simulink model "Simulink1potradi2"  (R2017b)
settings: Solver=VariableStepAuto  StartTime=0  StopTime=200  MinStep=0.1  RelTol=1e-3
values from neighbouring files (symbols this model uses):
  A = [0 1 1 1 ... (first row only)    [Initial.m]    (also in matlab_promjena_form.mat = [0 1 1 1 1 1 0 1 1 1 1 1 ... (25 elements, 5x5)])
  c_d = 2.5    [ardrone_params.m]    (also in matlab_promjena_form.mat)
  g = 9.81    [ardrone_params.m]    (also in matlab_promjena_form.mat)
  m = 1.65    [ardrone_params.m]    (also in matlab_promjena_form.mat)
  pitch_max = 0.4    [ardrone_params.m]    (also in matlab_promjena_form.mat)
  R1 = [0  -1  -1  -2  -2; 0  1  -1  2  -2]    [matlab_promjena_form.mat]
  R2 = [0,0,0,0; -1, 1, -3, 3]    [Initial.m]    (also in matlab_promjena_form.mat = [9  7  5  3  1; 0  0  0  0  0])
  roll_max = 0.4    [ardrone_params.m]    (also in matlab_promjena_form.mat)
  T_pitch = 0.4    [ardrone_params.m]    (also in matlab_promjena_form.mat)
  T_roll = 0.4    [ardrone_params.m]    (also in matlab_promjena_form.mat)
  T_yaw = 0.8    [ardrone_params.m]    (also in matlab_promjena_form.mat)
  T_z = 0.6    [ardrone_params.m]    (also in matlab_promjena_form.mat)
  x0 = [20, 60, 30, 50]    [Initial.m]    (also in matlab_promjena_form.mat = [0 -1 -1 -2 -2])
  y0 = [60, 20, 50, 30]    [Initial.m]    (also in matlab_promjena_form.mat = [0 1 -1 2 -2])
  yaw_rate_max = 0.7864    [ardrone_params.m]    (also in matlab_promjena_form.mat)
  z_rate_max = 0.7    [ardrone_params.m]    (also in matlab_promjena_form.mat)
settings Model: Creator=Mare  LastModifiedBy=Mare
settings SolverCC: ZeroCrossAlgorithm=Adaptive

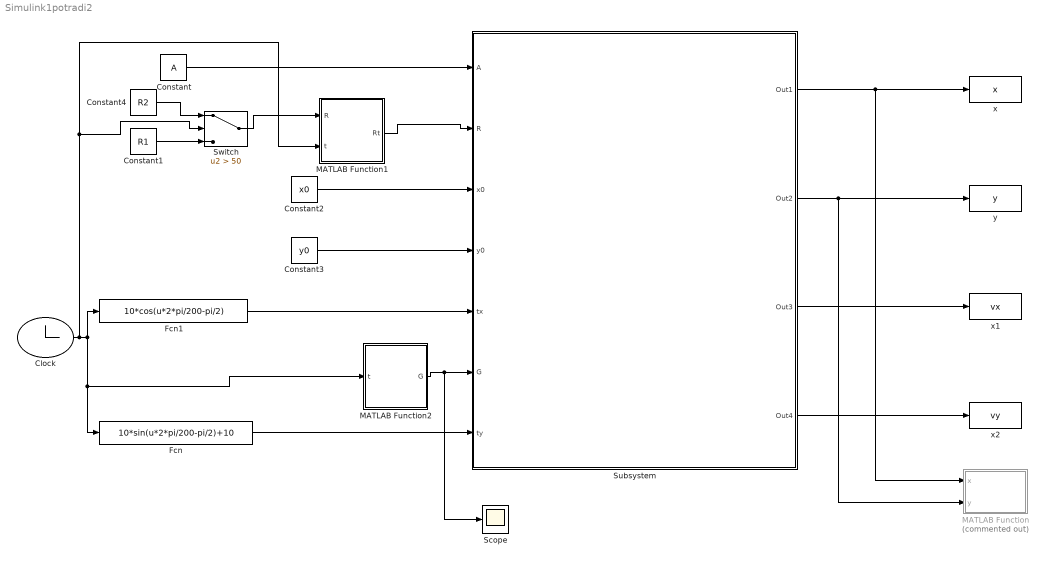
== system Simulink1potradi2 ==
  Clock : Clock
  Constant : Constant  Value=A
  Constant1 : Constant  Value=R1
  Constant2 : Constant  Value=x0
  Constant3 : Constant  Value=y0
  Constant4 : Constant  Value=R2
  Fcn : Fcn  Expr=10*sin(u*2*pi/200-pi/2)+10
  Fcn1 : Fcn  Expr=10*cos(u*2*pi/200-pi/2)
  MATLAB Function : MATLAB Function  Commented=on  TreatAsAtomicUnit=on
  MATLAB Function1 : MATLAB Function  TreatAsAtomicUnit=on
  MATLAB Function2 : MATLAB Function  TreatAsAtomicUnit=on
  Scope : Scope
  Subsystem : Subsystem
  Switch : Switch  Criteria=u2 > Threshold  Threshold=50
  x : ToWorkspace  VariableName=x  SaveFormat=Structure With Time  SampleTime=0.5
  x1 : ToWorkspace  VariableName=vx  SaveFormat=Structure With Time  SampleTime=0.5
  x2 : ToWorkspace  VariableName=vy  SaveFormat=Structure With Time  SampleTime=0.5
  y : ToWorkspace  VariableName=y  SaveFormat=Structure With Time  SampleTime=0.5
  wires:
  Subsystem/1(Out1) -> MATLAB Function/1(x), x/1
  Subsystem/2(Out2) -> MATLAB Function/2(y), y/1
  Constant3/1 -> Subsystem/4(y0)
  Constant2/1 -> Subsystem/3(x0)
  Constant1/1 -> Switch/3
  Constant/1 -> Subsystem/1(A)
  Subsystem/3(Out3) -> x1/1
  Subsystem/4(Out4) -> x2/1
  Clock/1 -> Switch/2, MATLAB Function1/2(t), Fcn1/1, MATLAB Function2/1(t), Fcn/1
  MATLAB Function2/1(G) -> Scope/1, Subsystem/6(G)
  MATLAB Function1/1(Rt) -> Subsystem/2(R)
  Fcn1/1 -> Subsystem/5(tx)
  Fcn/1 -> Subsystem/7(ty)
  Constant4/1 -> Switch/1
  Switch/1 -> MATLAB Function1/1(R)

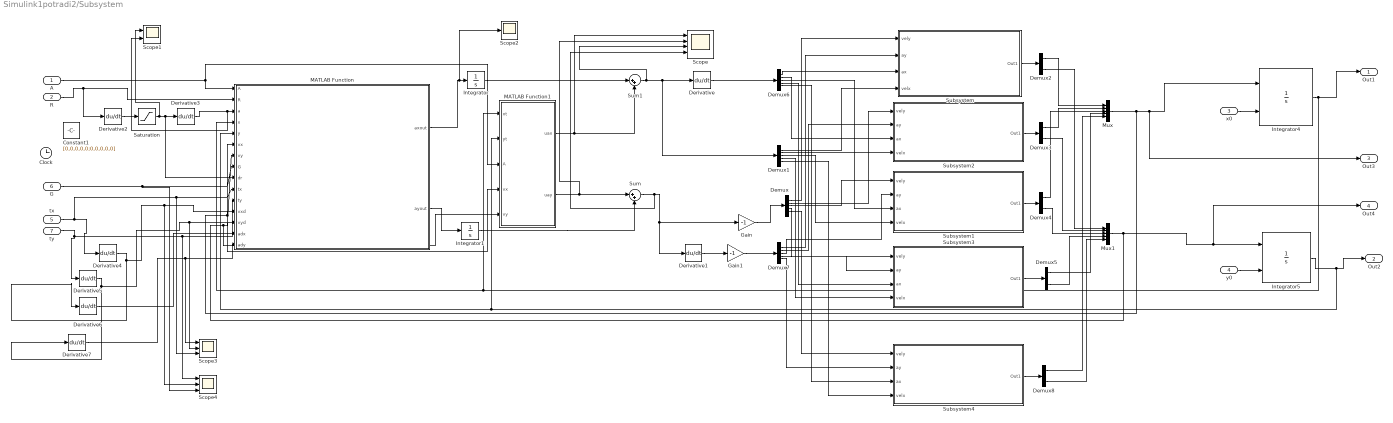
== system Simulink1potradi2/Subsystem ==
  A : Inport
  R : Inport  Port=2
  x0 : Inport  Port=3
  y0 : Inport  Port=4
  tx : Inport  Port=5
  G : Inport  Port=6
  ty : Inport  Port=7
  Clock : Clock
  Constant1 : Constant  Value=[0,0,0,0,0;0,0,0,0,0]
  Demux{,1,6..7} (4 alike) : Demux  Outputs=5
  Demux{2..5,8} (5 alike) : Demux  Outputs=2
  Derivative{,1..7} (8 alike) : Derivative
  Gain : Gain  Gain=-1
  Gain1 : Gain  Gain=-1
  Integrator : Integrator
  Integrator1 : Integrator
  Integrator4 : Integrator  InitialConditionSource=external
  Integrator5 : Integrator  InitialConditionSource=external
  MATLAB Function : MATLAB Function  TreatAsAtomicUnit=on
  MATLAB Function1 : MATLAB Function  TreatAsAtomicUnit=on
  Mux : Mux  Inputs=5
  Mux1 : Mux  Inputs=5
  Saturation : Saturate  UpperLimit=10000  LowerLimit=-10000
  Scope : Scope  NumInputPorts=4
  Scope1 : Scope  NumInputPorts=2
  Scope2 : Scope
  Scope3 : Scope  NumInputPorts=3
  Scope4 : Scope  NumInputPorts=3
  Subsystem : Subsystem
  Subsystem1 : Subsystem
  Subsystem2 : Subsystem
  Subsystem3 : Subsystem
  Subsystem4 : Subsystem
  Sum : Sum  Inputs=|++
  Sum1 : Sum  Inputs=|++
  Out1 : Outport
  Out2 : Outport  Port=2
  Out3 : Outport  Port=3
  Out4 : Outport  Port=4
  wires:
  A/1 -> MATLAB Function1/3(A), MATLAB Function/1(A)
  x0/1 -> Integrator4/2
  y0/1 -> Integrator5/2
  Integrator4/1 -> MATLAB Function1/1(xt), MATLAB Function/4(x), Out1/1
  Integrator5/1 -> MATLAB Function1/2(yt), MATLAB Function/5(y), Out2/1
  Demux1/1 -> Subsystem/4(velx)
  Demux1/2 -> Subsystem2/4(velx)
  Demux1/3 -> Subsystem1/4(velx)
  Demux/1 -> Subsystem/1("vely ")
  Demux/2 -> Subsystem2/1("vely ")
  Demux/3 -> Subsystem1/1("vely ")
  Demux1/4 -> Subsystem3/4(velx)
  Demux/4 -> Subsystem3/1("vely ")
  Subsystem/1(Out1) -> Demux2/1
  Subsystem2/1(Out1) -> Demux3/1
  Subsystem1/1(Out1) -> Demux4/1
  Subsystem3/1(Out1) -> Demux5/1
  Demux2/2 -> Mux1/1
  Demux2/1 -> Mux/1
  Demux3/1 -> Mux/2
  Demux4/1 -> Mux/3
  Demux5/1 -> Mux/4
  Demux3/2 -> Mux1/2
  Demux4/2 -> Mux1/3
  Demux5/2 -> Mux1/4
  Gain/1 -> Demux/1
  Demux6/1 -> Subsystem/3(ax)
  Demux6/2 -> Subsystem2/3(ax)
  Demux6/3 -> Subsystem1/3(ax)
  Demux6/4 -> Subsystem3/3(ax)
  Demux7/4 -> Subsystem3/2(ay)
  Demux7/3 -> Subsystem1/2(ay)
  Demux7/2 -> Subsystem2/2(ay)
  Demux7/1 -> Subsystem/2(ay)
  Gain1/1 -> Demux7/1
  MATLAB Function/1(axout) -> Scope2/1, Integrator/1
  Mux/1 -> MATLAB Function/6(vx), MATLAB Function1/4(vx), Out3/1, Integrator4/1
  Mux1/1 -> MATLAB Function1/5(vy), MATLAB Function/7(vy), Out4/1, Integrator5/1
  MATLAB Function1/2(uay) -> Scope/2, Sum/1
  MATLAB Function1/1(uax) -> Scope/1, Sum1/2
  Sum1/1 -> Scope/3, Demux1/1, Derivative/1
  Sum/1 -> Scope/4, Gain/1, Derivative1/1
  Integrator/1 -> Sum1/1
  Derivative/1 -> Demux6/1
  Derivative1/1 -> Gain1/1
  MATLAB Function/2(ayout) -> Integrator1/1
  Integrator1/1 -> Sum/2
  G/1 -> Scope4/3, MATLAB Function/8(G)
  Demux6/5 -> Subsystem4/3(ax)
  Demux1/5 -> Subsystem4/4(velx)
  Demux/5 -> Subsystem4/1("vely ")
  Demux7/5 -> Subsystem4/2(ay)
  Subsystem4/1(Out1) -> Demux8/1
  Demux8/1 -> Mux/5
  Demux8/2 -> Mux1/5
  tx/1 -> Scope3/3, MATLAB Function/10(tx), Derivative4/1
  ty/1 -> Scope4/1, MATLAB Function/11(ty), Derivative5/1
  R/1 -> Derivative2/1, MATLAB Function/2(R)
  Derivative2/1 -> Saturation/1
  Saturation/1 -> Scope1/1, MATLAB Function/9(dr), Derivative3/1
  Derivative3/1 -> Scope1/2, MATLAB Function/3(a)
  Derivative7/1 -> Scope3/1, MATLAB Function/15(ady)
  Derivative5/1 -> Derivative7/1, Scope3/2, MATLAB Function/13(vyd)
  Derivative4/1 -> Derivative6/1, Scope4/2, MATLAB Function/12(vxd)
  Derivative6/1 -> MATLAB Function/14(adx)

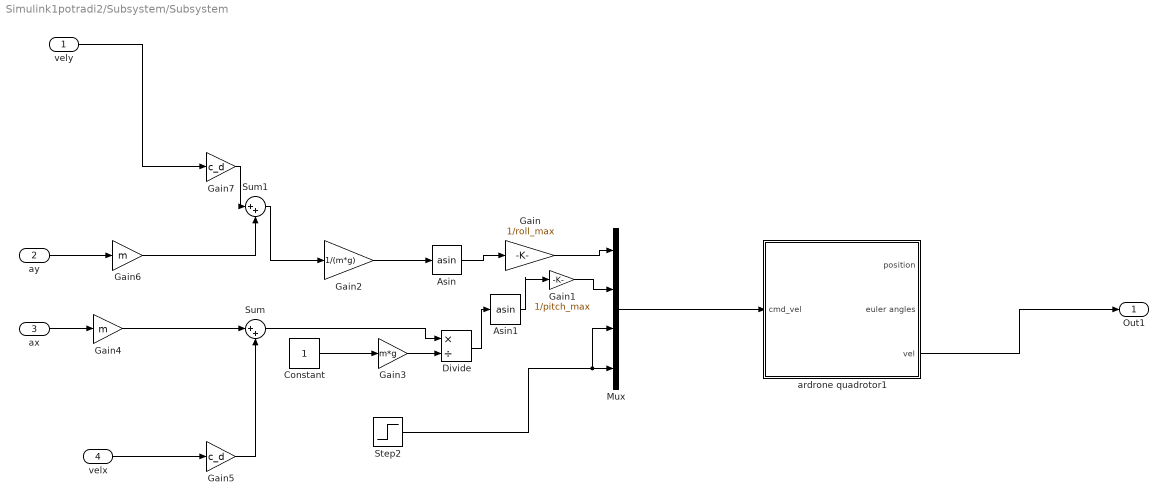
== system Simulink1potradi2/Subsystem/Subsystem ==
  "vely " : Inport
  ay : Inport  Port=2
  ax : Inport  Port=3
  velx : Inport  Port=4
  Asin : Trigonometry  Operator=asin
  Asin1 : Trigonometry  Operator=asin
  Constant : Constant
  Divide : Product  Inputs=*/
  Gain : Gain  Gain=1/roll_max
  Gain1 : Gain  Gain=1/pitch_max
  Gain2 : Gain  Gain=1/(m*g)
  Gain3 : Gain  Gain=m*g
  Gain4 : Gain  Gain=m
  Gain5 : Gain  Gain=c_d
  Gain6 : Gain  Gain=m
  Gain7 : Gain  Gain=c_d
  Mux : Mux
  Step2 : Step  Time=0  After=0  SampleTime=0
  Sum : Sum  Inputs=|++
  Sum1 : Sum  Inputs=|++
  ardrone quadrotor1 : Subsystem
  Out1 : Outport
  wires:
  Divide/1 -> Asin1/1
  ax/1 -> Gain4/1
  Gain4/1 -> Sum/1
  Constant/1 -> Gain3/1
  Gain5/1 -> Sum/2
  Mux/1 -> ardrone quadrotor1/1(cmd_vel)
  Asin/1 -> Gain/1
  Step2/1 -> Mux/3, Mux/4
  Sum1/1 -> Gain2/1
  Gain2/1 -> Asin/1
  ay/1 -> Gain6/1
  Gain6/1 -> Sum1/2
  Gain3/1 -> Divide/2
  "vely "/1 -> Gain7/1
  velx/1 -> Gain5/1
  Gain7/1 -> Sum1/1
  Asin1/1 -> Gain1/1
  Sum/1 -> Divide/1
  ardrone quadrotor1/3(vel) -> Out1/1
  Gain/1 -> Mux/1
  Gain1/1 -> Mux/2

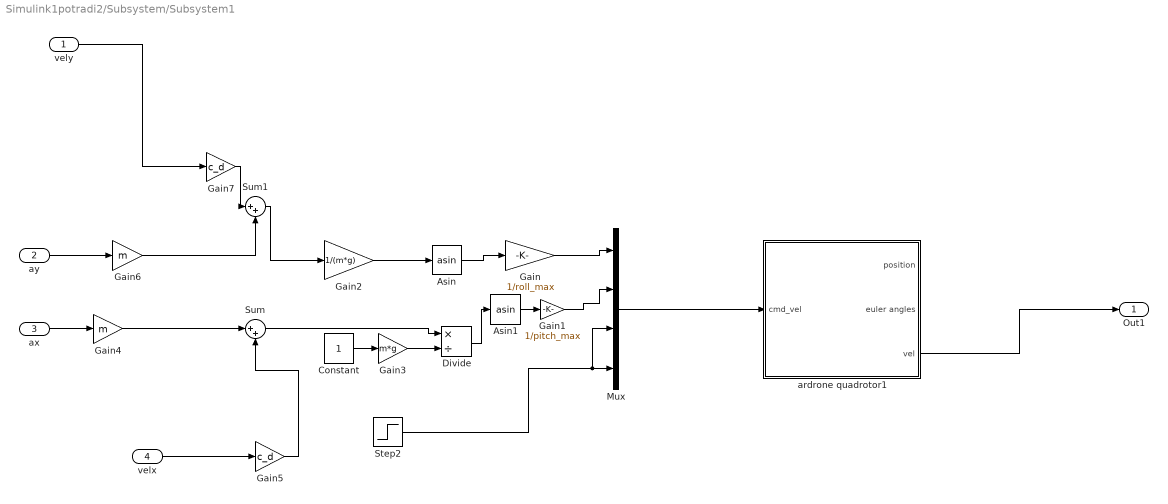
== system Simulink1potradi2/Subsystem/Subsystem1 ==
  "vely " : Inport
  ay : Inport  Port=2
  ax : Inport  Port=3
  velx : Inport  Port=4
  Asin : Trigonometry  Operator=asin
  Asin1 : Trigonometry  Operator=asin
  Constant : Constant
  Divide : Product  Inputs=*/
  Gain : Gain  Gain=1/roll_max
  Gain1 : Gain  Gain=1/pitch_max
  Gain2 : Gain  Gain=1/(m*g)
  Gain3 : Gain  Gain=m*g
  Gain4 : Gain  Gain=m
  Gain5 : Gain  Gain=c_d
  Gain6 : Gain  Gain=m
  Gain7 : Gain  Gain=c_d
  Mux : Mux
  Step2 : Step  Time=0  After=0  SampleTime=0
  Sum : Sum  Inputs=|++
  Sum1 : Sum  Inputs=|++
  ardrone quadrotor1 : Subsystem
  Out1 : Outport
  wires:
  Divide/1 -> Asin1/1
  ax/1 -> Gain4/1
  Gain4/1 -> Sum/1
  Constant/1 -> Gain3/1
  Gain5/1 -> Sum/2
  Mux/1 -> ardrone quadrotor1/1(cmd_vel)
  Asin/1 -> Gain/1
  Step2/1 -> Mux/3, Mux/4
  Sum1/1 -> Gain2/1
  Gain2/1 -> Asin/1
  ay/1 -> Gain6/1
  Gain6/1 -> Sum1/2
  Gain3/1 -> Divide/2
  "vely "/1 -> Gain7/1
  velx/1 -> Gain5/1
  Gain7/1 -> Sum1/1
  Asin1/1 -> Gain1/1
  Sum/1 -> Divide/1
  ardrone quadrotor1/3(vel) -> Out1/1
  Gain/1 -> Mux/1
  Gain1/1 -> Mux/2

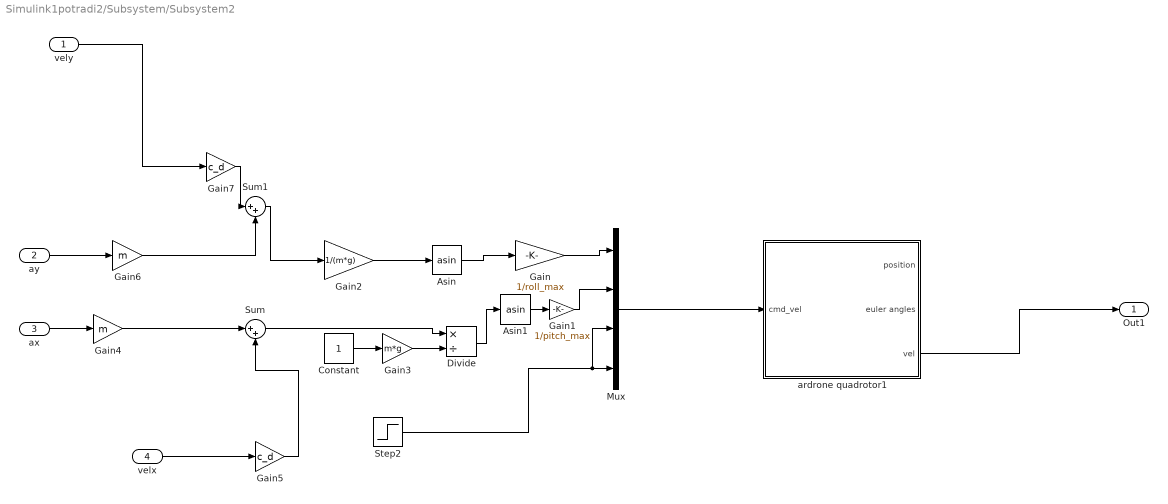
== system Simulink1potradi2/Subsystem/Subsystem2 ==
  "vely " : Inport
  ay : Inport  Port=2
  ax : Inport  Port=3
  velx : Inport  Port=4
  Asin : Trigonometry  Operator=asin
  Asin1 : Trigonometry  Operator=asin
  Constant : Constant
  Divide : Product  Inputs=*/
  Gain : Gain  Gain=1/roll_max
  Gain1 : Gain  Gain=1/pitch_max
  Gain2 : Gain  Gain=1/(m*g)
  Gain3 : Gain  Gain=m*g
  Gain4 : Gain  Gain=m
  Gain5 : Gain  Gain=c_d
  Gain6 : Gain  Gain=m
  Gain7 : Gain  Gain=c_d
  Mux : Mux
  Step2 : Step  Time=0  After=0  SampleTime=0
  Sum : Sum  Inputs=|++
  Sum1 : Sum  Inputs=|++
  ardrone quadrotor1 : Subsystem
  Out1 : Outport
  wires:
  Divide/1 -> Asin1/1
  ax/1 -> Gain4/1
  Gain4/1 -> Sum/1
  Constant/1 -> Gain3/1
  Gain5/1 -> Sum/2
  Mux/1 -> ardrone quadrotor1/1(cmd_vel)
  Asin/1 -> Gain/1
  Step2/1 -> Mux/3, Mux/4
  Sum1/1 -> Gain2/1
  Gain2/1 -> Asin/1
  ay/1 -> Gain6/1
  Gain6/1 -> Sum1/2
  Gain3/1 -> Divide/2
  "vely "/1 -> Gain7/1
  velx/1 -> Gain5/1
  Gain7/1 -> Sum1/1
  Asin1/1 -> Gain1/1
  Sum/1 -> Divide/1
  ardrone quadrotor1/3(vel) -> Out1/1
  Gain/1 -> Mux/1
  Gain1/1 -> Mux/2

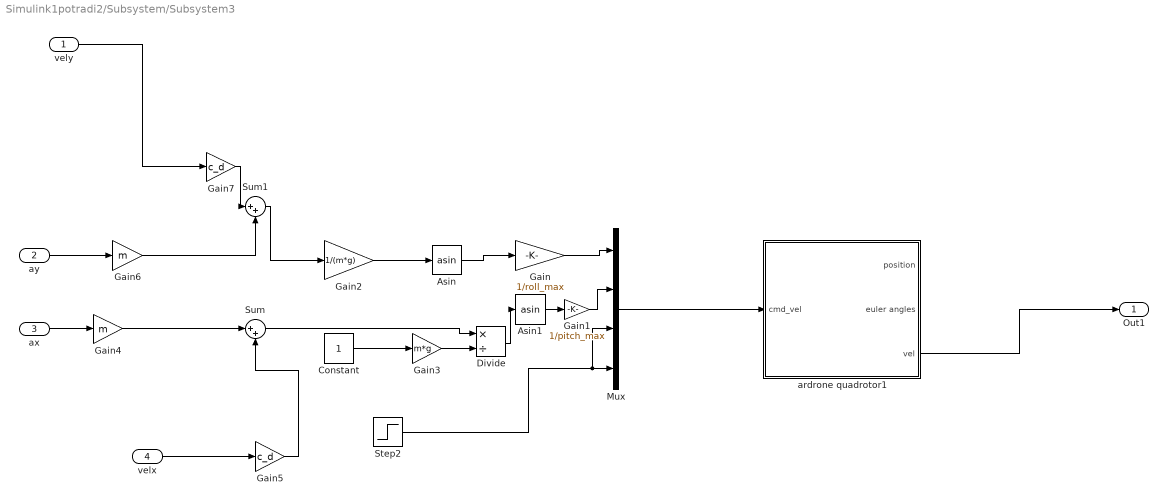
== system Simulink1potradi2/Subsystem/Subsystem3 ==
  "vely " : Inport
  ay : Inport  Port=2
  ax : Inport  Port=3
  velx : Inport  Port=4
  Asin : Trigonometry  Operator=asin
  Asin1 : Trigonometry  Operator=asin
  Constant : Constant
  Divide : Product  Inputs=*/
  Gain : Gain  Gain=1/roll_max
  Gain1 : Gain  Gain=1/pitch_max
  Gain2 : Gain  Gain=1/(m*g)
  Gain3 : Gain  Gain=m*g
  Gain4 : Gain  Gain=m
  Gain5 : Gain  Gain=c_d
  Gain6 : Gain  Gain=m
  Gain7 : Gain  Gain=c_d
  Mux : Mux
  Step2 : Step  Time=0  After=0  SampleTime=0
  Sum : Sum  Inputs=|++
  Sum1 : Sum  Inputs=|++
  ardrone quadrotor1 : Subsystem
  Out1 : Outport
  wires:
  Divide/1 -> Asin1/1
  ax/1 -> Gain4/1
  Gain4/1 -> Sum/1
  Constant/1 -> Gain3/1
  Gain5/1 -> Sum/2
  Mux/1 -> ardrone quadrotor1/1(cmd_vel)
  Asin/1 -> Gain/1
  Step2/1 -> Mux/3, Mux/4
  Sum1/1 -> Gain2/1
  Gain2/1 -> Asin/1
  ay/1 -> Gain6/1
  Gain6/1 -> Sum1/2
  Gain3/1 -> Divide/2
  "vely "/1 -> Gain7/1
  velx/1 -> Gain5/1
  Gain7/1 -> Sum1/1
  Asin1/1 -> Gain1/1
  Sum/1 -> Divide/1
  ardrone quadrotor1/3(vel) -> Out1/1
  Gain/1 -> Mux/1
  Gain1/1 -> Mux/2

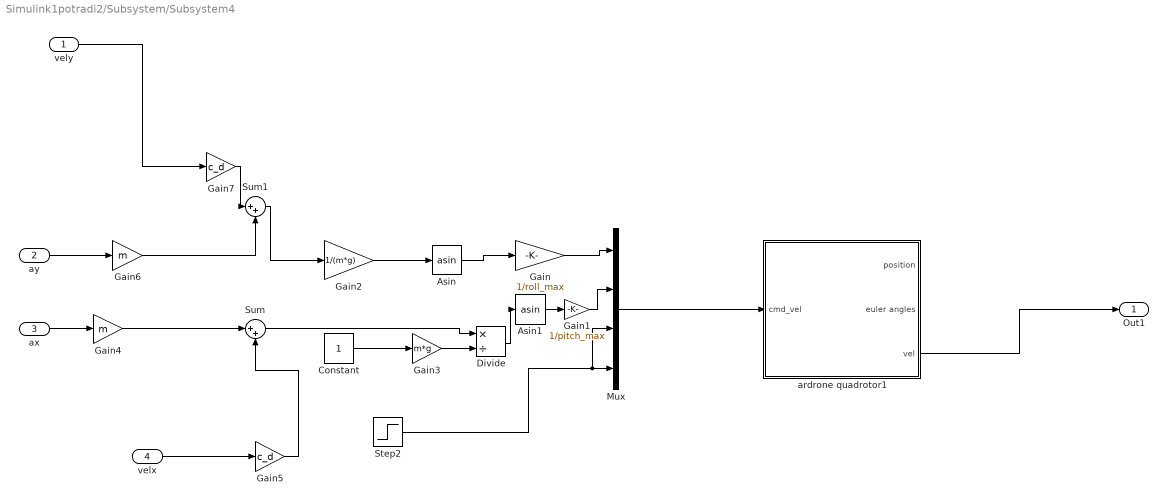
== system Simulink1potradi2/Subsystem/Subsystem4 ==
  "vely " : Inport
  ay : Inport  Port=2
  ax : Inport  Port=3
  velx : Inport  Port=4
  Asin : Trigonometry  Operator=asin
  Asin1 : Trigonometry  Operator=asin
  Constant : Constant
  Divide : Product  Inputs=*/
  Gain : Gain  Gain=1/roll_max
  Gain1 : Gain  Gain=1/pitch_max
  Gain2 : Gain  Gain=1/(m*g)
  Gain3 : Gain  Gain=m*g
  Gain4 : Gain  Gain=m
  Gain5 : Gain  Gain=c_d
  Gain6 : Gain  Gain=m
  Gain7 : Gain  Gain=c_d
  Mux : Mux
  Step2 : Step  Time=0  After=0  SampleTime=0
  Sum : Sum  Inputs=|++
  Sum1 : Sum  Inputs=|++
  ardrone quadrotor1 : Subsystem
  Out1 : Outport
  wires:
  Divide/1 -> Asin1/1
  ax/1 -> Gain4/1
  Gain4/1 -> Sum/1
  Constant/1 -> Gain3/1
  Gain5/1 -> Sum/2
  Mux/1 -> ardrone quadrotor1/1(cmd_vel)
  Asin/1 -> Gain/1
  Step2/1 -> Mux/3, Mux/4
  Sum1/1 -> Gain2/1
  Gain2/1 -> Asin/1
  ay/1 -> Gain6/1
  Gain6/1 -> Sum1/2
  Gain3/1 -> Divide/2
  "vely "/1 -> Gain7/1
  velx/1 -> Gain5/1
  Gain7/1 -> Sum1/1
  Asin1/1 -> Gain1/1
  Sum/1 -> Divide/1
  ardrone quadrotor1/3(vel) -> Out1/1
  Gain/1 -> Mux/1
  Gain1/1 -> Mux/2

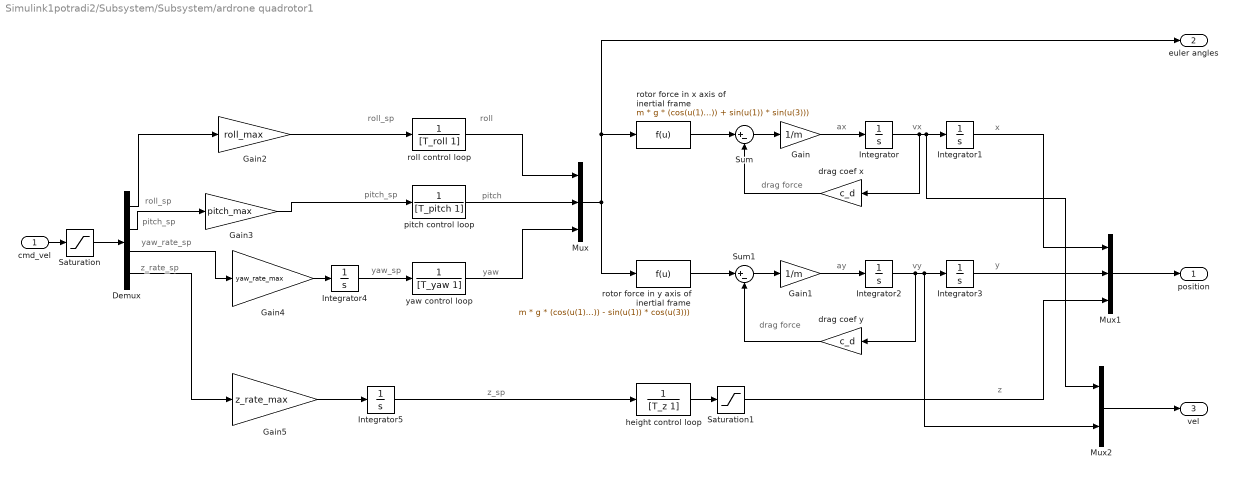
== system Simulink1potradi2/Subsystem/Subsystem/ardrone quadrotor1 ==
  note: pitch_sp
  note: roll_sp
  note: z_sp
  note: yaw_sp
  note: pitch_sp
  note: roll_sp
  note: z
  note: y
  note: x
  note: z_rate_sp
  note: yaw_rate_sp
  note: drag force
  note: drag force
  note: vx
  note: ax
  note: yaw
  note: pitch
  note: roll
  note: vy
  note: ay
  cmd_vel : Inport
  Demux : Demux
  Gain : Gain  Gain=1/m
  Gain1 : Gain  Gain=1/m
  Gain2 : Gain  Gain=roll_max
  Gain3 : Gain  Gain=pitch_max
  Gain4 : Gain  Gain=yaw_rate_max
  Gain5 : Gain  Gain=z_rate_max
  Integrator{,1..5} (6 alike) : Integrator
  Mux : Mux  Inputs=3
  Mux1 : Mux  Inputs=3
  Mux2 : Mux  Inputs=2
  Saturation : Saturate  UpperLimit=1  LowerLimit=-1
  Saturation1 : Saturate  UpperLimit=Inf  LowerLimit=0
  Sum : Sum  Inputs=|+-
  Sum1 : Sum  Inputs=|+-
  drag coef x : Gain  Gain=c_d
  drag coef y : Gain  Gain=c_d
  height control loop : TransferFcn  Denominator=[T_z 1]
  pitch control loop : TransferFcn  Denominator=[T_pitch 1]
  roll control loop : TransferFcn  Denominator=[T_roll 1]
  rotor force in x axis of inertial frame : Fcn  Expr=m * g * (cos(u(1)) * sin(u(2)) * cos (u(3)) + sin(u(1)) * sin(u(3)))
  rotor force in y axis of inertial frame : Fcn  Expr=m * g * (cos(u(1)) * sin(u(2)) * sin (u(3)) - sin(u(1)) * cos(u(3)))
  yaw control loop : TransferFcn  Denominator=[T_yaw 1]
  position : Outport
  euler angles : Outport  Port=2
  vel : Outport  Port=3
  wires:
  Gain1/1 -> Integrator2/1
  Integrator2/1 -> drag coef y/1, Mux2/2, Integrator3/1
  drag coef x/1 -> Sum/2
  Mux/1 -> rotor force in y axis of inertial frame/1, euler angles/1, rotor force in x axis of inertial frame/1
  pitch control loop/1 -> Mux/2
  yaw control loop/1 -> Mux/3
  rotor force in y axis of inertial frame/1 -> Sum1/1
  Sum/1 -> Gain/1
  roll control loop/1 -> Mux/1
  rotor force in x axis of inertial frame/1 -> Sum/1
  drag coef y/1 -> Sum1/2
  Gain/1 -> Integrator/1
  Sum1/1 -> Gain1/1
  Demux/3 -> Gain4/1
  Demux/4 -> Gain5/1
  Integrator1/1 -> Mux1/1
  Integrator3/1 -> Mux1/2
  height control loop/1 -> Saturation1/1
  Mux1/1 -> position/1
  Integrator/1 -> drag coef x/1, Mux2/1, Integrator1/1
  Demux/1 -> Gain2/1
  Demux/2 -> Gain3/1
  Integrator4/1 -> yaw control loop/1
  Gain4/1 -> Integrator4/1
  Gain5/1 -> Integrator5/1
  Integrator5/1 -> height control loop/1
  cmd_vel/1 -> Saturation/1
  Saturation1/1 -> Mux1/3
  Mux2/1 -> vel/1
  Saturation/1 -> Demux/1
  Gain2/1 -> roll control loop/1
  Gain3/1 -> pitch control loop/1

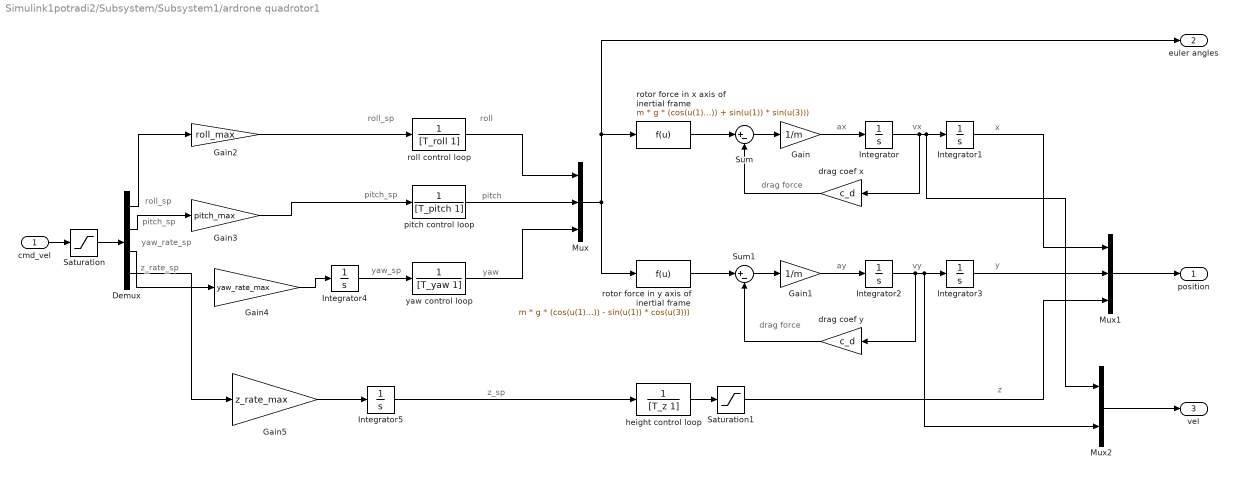
== system Simulink1potradi2/Subsystem/Subsystem1/ardrone quadrotor1 ==
  note: pitch_sp
  note: roll_sp
  note: z_sp
  note: yaw_sp
  note: pitch_sp
  note: roll_sp
  note: z
  note: y
  note: x
  note: z_rate_sp
  note: yaw_rate_sp
  note: drag force
  note: drag force
  note: vx
  note: ax
  note: yaw
  note: pitch
  note: roll
  note: vy
  note: ay
  cmd_vel : Inport
  Demux : Demux
  Gain : Gain  Gain=1/m
  Gain1 : Gain  Gain=1/m
  Gain2 : Gain  Gain=roll_max
  Gain3 : Gain  Gain=pitch_max
  Gain4 : Gain  Gain=yaw_rate_max
  Gain5 : Gain  Gain=z_rate_max
  Integrator{,1..5} (6 alike) : Integrator
  Mux : Mux  Inputs=3
  Mux1 : Mux  Inputs=3
  Mux2 : Mux  Inputs=2
  Saturation : Saturate  UpperLimit=1  LowerLimit=-1
  Saturation1 : Saturate  UpperLimit=Inf  LowerLimit=0
  Sum : Sum  Inputs=|+-
  Sum1 : Sum  Inputs=|+-
  drag coef x : Gain  Gain=c_d
  drag coef y : Gain  Gain=c_d
  height control loop : TransferFcn  Denominator=[T_z 1]
  pitch control loop : TransferFcn  Denominator=[T_pitch 1]
  roll control loop : TransferFcn  Denominator=[T_roll 1]
  rotor force in x axis of inertial frame : Fcn  Expr=m * g * (cos(u(1)) * sin(u(2)) * cos (u(3)) + sin(u(1)) * sin(u(3)))
  rotor force in y axis of inertial frame : Fcn  Expr=m * g * (cos(u(1)) * sin(u(2)) * sin (u(3)) - sin(u(1)) * cos(u(3)))
  yaw control loop : TransferFcn  Denominator=[T_yaw 1]
  position : Outport
  euler angles : Outport  Port=2
  vel : Outport  Port=3
  wires:
  Gain1/1 -> Integrator2/1
  Integrator2/1 -> drag coef y/1, Mux2/2, Integrator3/1
  drag coef x/1 -> Sum/2
  Mux/1 -> rotor force in y axis of inertial frame/1, euler angles/1, rotor force in x axis of inertial frame/1
  pitch control loop/1 -> Mux/2
  yaw control loop/1 -> Mux/3
  rotor force in y axis of inertial frame/1 -> Sum1/1
  Sum/1 -> Gain/1
  roll control loop/1 -> Mux/1
  rotor force in x axis of inertial frame/1 -> Sum/1
  drag coef y/1 -> Sum1/2
  Gain/1 -> Integrator/1
  Sum1/1 -> Gain1/1
  Demux/4 -> Gain5/1
  Integrator1/1 -> Mux1/1
  Integrator3/1 -> Mux1/2
  height control loop/1 -> Saturation1/1
  Mux1/1 -> position/1
  Integrator/1 -> drag coef x/1, Mux2/1, Integrator1/1
  Demux/1 -> Gain2/1
  Demux/2 -> Gain3/1
  Integrator4/1 -> yaw control loop/1
  Demux/3 -> Gain4/1
  Gain5/1 -> Integrator5/1
  Integrator5/1 -> height control loop/1
  cmd_vel/1 -> Saturation/1
  Saturation1/1 -> Mux1/3
  Mux2/1 -> vel/1
  Saturation/1 -> Demux/1
  Gain2/1 -> roll control loop/1
  Gain3/1 -> pitch control loop/1
  Gain4/1 -> Integrator4/1

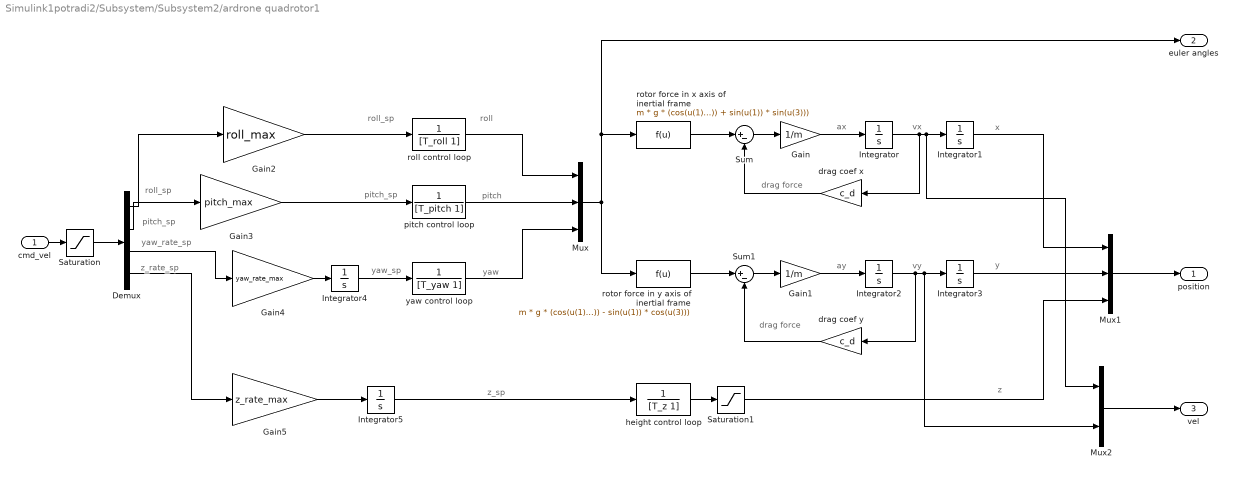
== system Simulink1potradi2/Subsystem/Subsystem2/ardrone quadrotor1 ==
  note: pitch_sp
  note: roll_sp
  note: z_sp
  note: yaw_sp
  note: pitch_sp
  note: roll_sp
  note: z
  note: y
  note: x
  note: z_rate_sp
  note: yaw_rate_sp
  note: drag force
  note: drag force
  note: vx
  note: ax
  note: yaw
  note: pitch
  note: roll
  note: vy
  note: ay
  cmd_vel : Inport
  Demux : Demux
  Gain : Gain  Gain=1/m
  Gain1 : Gain  Gain=1/m
  Gain2 : Gain  Gain=roll_max
  Gain3 : Gain  Gain=pitch_max
  Gain4 : Gain  Gain=yaw_rate_max
  Gain5 : Gain  Gain=z_rate_max
  Integrator{,1..5} (6 alike) : Integrator
  Mux : Mux  Inputs=3
  Mux1 : Mux  Inputs=3
  Mux2 : Mux  Inputs=2
  Saturation : Saturate  UpperLimit=1  LowerLimit=-1
  Saturation1 : Saturate  UpperLimit=Inf  LowerLimit=0
  Sum : Sum  Inputs=|+-
  Sum1 : Sum  Inputs=|+-
  drag coef x : Gain  Gain=c_d
  drag coef y : Gain  Gain=c_d
  height control loop : TransferFcn  Denominator=[T_z 1]
  pitch control loop : TransferFcn  Denominator=[T_pitch 1]
  roll control loop : TransferFcn  Denominator=[T_roll 1]
  rotor force in x axis of inertial frame : Fcn  Expr=m * g * (cos(u(1)) * sin(u(2)) * cos (u(3)) + sin(u(1)) * sin(u(3)))
  rotor force in y axis of inertial frame : Fcn  Expr=m * g * (cos(u(1)) * sin(u(2)) * sin (u(3)) - sin(u(1)) * cos(u(3)))
  yaw control loop : TransferFcn  Denominator=[T_yaw 1]
  position : Outport
  euler angles : Outport  Port=2
  vel : Outport  Port=3
  wires:
  Gain1/1 -> Integrator2/1
  Integrator2/1 -> drag coef y/1, Mux2/2, Integrator3/1
  drag coef x/1 -> Sum/2
  Mux/1 -> rotor force in y axis of inertial frame/1, euler angles/1, rotor force in x axis of inertial frame/1
  pitch control loop/1 -> Mux/2
  yaw control loop/1 -> Mux/3
  rotor force in y axis of inertial frame/1 -> Sum1/1
  Sum/1 -> Gain/1
  roll control loop/1 -> Mux/1
  rotor force in x axis of inertial frame/1 -> Sum/1
  drag coef y/1 -> Sum1/2
  Gain/1 -> Integrator/1
  Sum1/1 -> Gain1/1
  Demux/3 -> Gain4/1
  Demux/4 -> Gain5/1
  Integrator1/1 -> Mux1/1
  Integrator3/1 -> Mux1/2
  height control loop/1 -> Saturation1/1
  Mux1/1 -> position/1
  Integrator/1 -> drag coef x/1, Mux2/1, Integrator1/1
  Demux/1 -> Gain2/1
  Demux/2 -> Gain3/1
  Integrator4/1 -> yaw control loop/1
  Gain4/1 -> Integrator4/1
  Gain5/1 -> Integrator5/1
  Integrator5/1 -> height control loop/1
  cmd_vel/1 -> Saturation/1
  Saturation1/1 -> Mux1/3
  Mux2/1 -> vel/1
  Saturation/1 -> Demux/1
  Gain2/1 -> roll control loop/1
  Gain3/1 -> pitch control loop/1

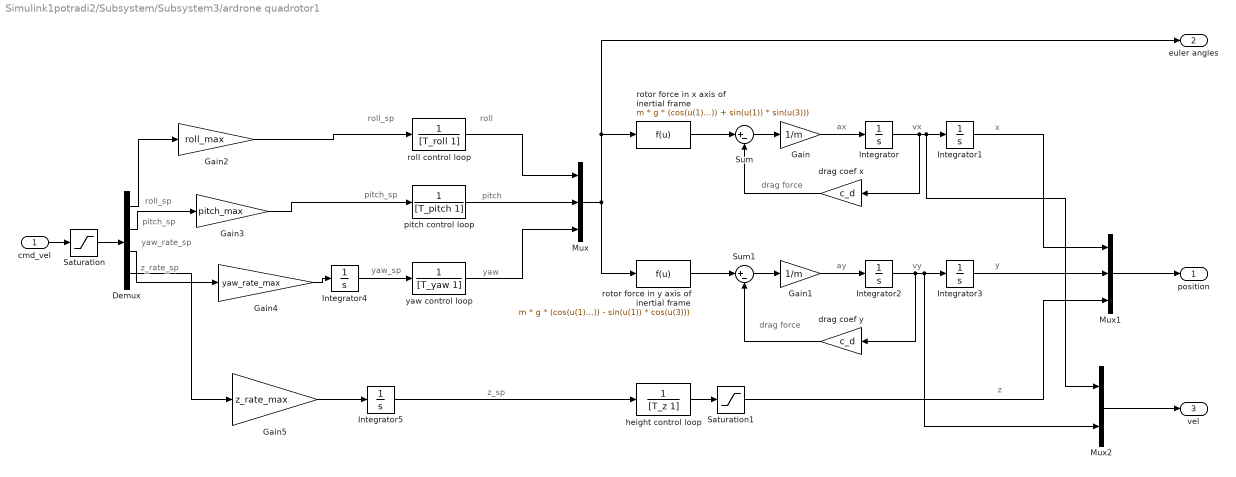
== system Simulink1potradi2/Subsystem/Subsystem3/ardrone quadrotor1 ==
  note: pitch_sp
  note: roll_sp
  note: z_sp
  note: yaw_sp
  note: pitch_sp
  note: roll_sp
  note: z
  note: y
  note: x
  note: z_rate_sp
  note: yaw_rate_sp
  note: drag force
  note: drag force
  note: vx
  note: ax
  note: yaw
  note: pitch
  note: roll
  note: vy
  note: ay
  cmd_vel : Inport
  Demux : Demux
  Gain : Gain  Gain=1/m
  Gain1 : Gain  Gain=1/m
  Gain2 : Gain  Gain=roll_max
  Gain3 : Gain  Gain=pitch_max
  Gain4 : Gain  Gain=yaw_rate_max
  Gain5 : Gain  Gain=z_rate_max
  Integrator{,1..5} (6 alike) : Integrator
  Mux : Mux  Inputs=3
  Mux1 : Mux  Inputs=3
  Mux2 : Mux  Inputs=2
  Saturation : Saturate  UpperLimit=1  LowerLimit=-1
  Saturation1 : Saturate  UpperLimit=Inf  LowerLimit=0
  Sum : Sum  Inputs=|+-
  Sum1 : Sum  Inputs=|+-
  drag coef x : Gain  Gain=c_d
  drag coef y : Gain  Gain=c_d
  height control loop : TransferFcn  Denominator=[T_z 1]
  pitch control loop : TransferFcn  Denominator=[T_pitch 1]
  roll control loop : TransferFcn  Denominator=[T_roll 1]
  rotor force in x axis of inertial frame : Fcn  Expr=m * g * (cos(u(1)) * sin(u(2)) * cos (u(3)) + sin(u(1)) * sin(u(3)))
  rotor force in y axis of inertial frame : Fcn  Expr=m * g * (cos(u(1)) * sin(u(2)) * sin (u(3)) - sin(u(1)) * cos(u(3)))
  yaw control loop : TransferFcn  Denominator=[T_yaw 1]
  position : Outport
  euler angles : Outport  Port=2
  vel : Outport  Port=3
  wires:
  Gain1/1 -> Integrator2/1
  Integrator2/1 -> drag coef y/1, Mux2/2, Integrator3/1
  drag coef x/1 -> Sum/2
  Mux/1 -> rotor force in y axis of inertial frame/1, euler angles/1, rotor force in x axis of inertial frame/1
  pitch control loop/1 -> Mux/2
  yaw control loop/1 -> Mux/3
  rotor force in y axis of inertial frame/1 -> Sum1/1
  Sum/1 -> Gain/1
  roll control loop/1 -> Mux/1
  rotor force in x axis of inertial frame/1 -> Sum/1
  drag coef y/1 -> Sum1/2
  Gain/1 -> Integrator/1
  Sum1/1 -> Gain1/1
  Demux/4 -> Gain5/1
  Integrator1/1 -> Mux1/1
  Integrator3/1 -> Mux1/2
  height control loop/1 -> Saturation1/1
  Mux1/1 -> position/1
  Integrator/1 -> drag coef x/1, Mux2/1, Integrator1/1
  Demux/1 -> Gain2/1
  Demux/2 -> Gain3/1
  Integrator4/1 -> yaw control loop/1
  Demux/3 -> Gain4/1
  Gain5/1 -> Integrator5/1
  Integrator5/1 -> height control loop/1
  cmd_vel/1 -> Saturation/1
  Saturation1/1 -> Mux1/3
  Mux2/1 -> vel/1
  Saturation/1 -> Demux/1
  Gain2/1 -> roll control loop/1
  Gain3/1 -> pitch control loop/1
  Gain4/1 -> Integrator4/1

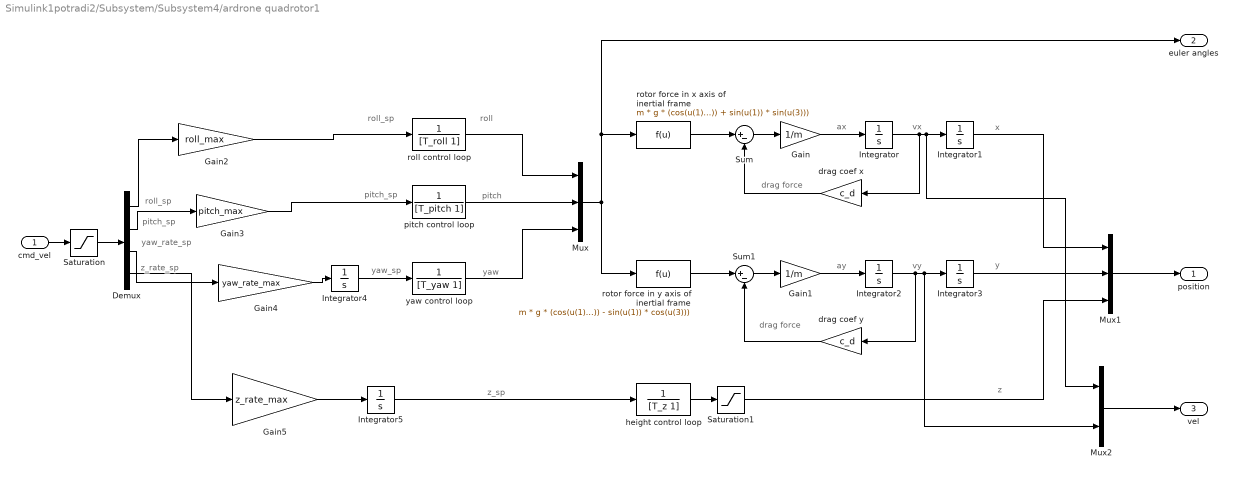
== system Simulink1potradi2/Subsystem/Subsystem4/ardrone quadrotor1 ==
  note: pitch_sp
  note: roll_sp
  note: z_sp
  note: yaw_sp
  note: pitch_sp
  note: roll_sp
  note: z
  note: y
  note: x
  note: z_rate_sp
  note: yaw_rate_sp
  note: drag force
  note: drag force
  note: vx
  note: ax
  note: yaw
  note: pitch
  note: roll
  note: vy
  note: ay
  cmd_vel : Inport
  Demux : Demux
  Gain : Gain  Gain=1/m
  Gain1 : Gain  Gain=1/m
  Gain2 : Gain  Gain=roll_max
  Gain3 : Gain  Gain=pitch_max
  Gain4 : Gain  Gain=yaw_rate_max
  Gain5 : Gain  Gain=z_rate_max
  Integrator{,1..5} (6 alike) : Integrator
  Mux : Mux  Inputs=3
  Mux1 : Mux  Inputs=3
  Mux2 : Mux  Inputs=2
  Saturation : Saturate  UpperLimit=1  LowerLimit=-1
  Saturation1 : Saturate  UpperLimit=Inf  LowerLimit=0
  Sum : Sum  Inputs=|+-
  Sum1 : Sum  Inputs=|+-
  drag coef x : Gain  Gain=c_d
  drag coef y : Gain  Gain=c_d
  height control loop : TransferFcn  Denominator=[T_z 1]
  pitch control loop : TransferFcn  Denominator=[T_pitch 1]
  roll control loop : TransferFcn  Denominator=[T_roll 1]
  rotor force in x axis of inertial frame : Fcn  Expr=m * g * (cos(u(1)) * sin(u(2)) * cos (u(3)) + sin(u(1)) * sin(u(3)))
  rotor force in y axis of inertial frame : Fcn  Expr=m * g * (cos(u(1)) * sin(u(2)) * sin (u(3)) - sin(u(1)) * cos(u(3)))
  yaw control loop : TransferFcn  Denominator=[T_yaw 1]
  position : Outport
  euler angles : Outport  Port=2
  vel : Outport  Port=3
  wires:
  Gain1/1 -> Integrator2/1
  Integrator2/1 -> drag coef y/1, Mux2/2, Integrator3/1
  drag coef x/1 -> Sum/2
  Mux/1 -> rotor force in y axis of inertial frame/1, euler angles/1, rotor force in x axis of inertial frame/1
  pitch control loop/1 -> Mux/2
  yaw control loop/1 -> Mux/3
  rotor force in y axis of inertial frame/1 -> Sum1/1
  Sum/1 -> Gain/1
  roll control loop/1 -> Mux/1
  rotor force in x axis of inertial frame/1 -> Sum/1
  drag coef y/1 -> Sum1/2
  Gain/1 -> Integrator/1
  Sum1/1 -> Gain1/1
  Demux/4 -> Gain5/1
  Integrator1/1 -> Mux1/1
  Integrator3/1 -> Mux1/2
  height control loop/1 -> Saturation1/1
  Mux1/1 -> position/1
  Integrator/1 -> drag coef x/1, Mux2/1, Integrator1/1
  Demux/1 -> Gain2/1
  Demux/2 -> Gain3/1
  Integrator4/1 -> yaw control loop/1
  Demux/3 -> Gain4/1
  Gain5/1 -> Integrator5/1
  Integrator5/1 -> height control loop/1
  cmd_vel/1 -> Saturation/1
  Saturation1/1 -> Mux1/3
  Mux2/1 -> vel/1
  Saturation/1 -> Demux/1
  Gain2/1 -> roll control loop/1
  Gain3/1 -> pitch control loop/1
  Gain4/1 -> Integrator4/1

== matlab function Simulink1potradi2/Subsystem/MATLAB Function ==
  data: axout output; A input; ayout output; R input; a input; x input; y input; vx input; vy input; G input; dr input; tx input; ty input; vxd input; vyd input; adx input; ady input
function [axout,ayout]= fcn(A, R, a ,x,y,vx,vy, G, dr, tx,ty,vxd,vyd, adx, ady)
axout=zeros(1,length(A));
ayout = zeros(1, length(A));
%azout = zeros(length(A),1);
beta = 0.05;
gama = 38;

% xc = 0;
% yc = 0;


for i = 1:length(A)
    axout(i) = (a(1,i)+adx - beta*(x(i)-(R(1,i)+tx)) - gama*beta*(vx(i)-dr(1,i)-vxd));
    ayout(i) = (a(2,i)+ady - beta*(y(i)-(R(2,i)+ty)) - gama*beta*(vy(i)-dr(2,i)-vyd));
    %azout(i) = 0 - C(i)*vz(i);
    for j = 1:length(A)
        axout(i) = axout(i) - G(i,j)*A(i,j)*((x(i)-R(1,i))-(x(j)-R(1,j))+ gama*((vx(i)-dr(1,i))-(vx(j)-dr(1,j))));
        ayout(i) = ayout(i) - G(i,j)*A(i,j)*((y(i)-R(2,i))-(y(j)-R(2,j))+ gama*((vy(i)-dr(2,i))-(vy(j)-dr(2,j))));
        %azout(i) = azout(i) - A(i,j)*(B(j)*(z(i)-R(3,i))-(y(j)-R(3,j))+ C(j)*(vz(i)-vz(j)));
    end
end

== matlab function Simulink1potradi2/MATLAB Function ==
  data: x input; y input
function  fcn(x,y)
%postavljanje granicnih vrijednosti koordinata
xmax = 25;
xmin = -25;
ymax = 25;
ymin = -10;

colors = {[0.6,0.9,0.6],[0,0.7,1],[0.85, 0.6,0.85],[1,0.8,0],[0.9,0.6,0.5], [0,1,0],[1,0,0]};


cla;
axis([xmin,xmax,ymin,ymax]);
xlabel('x');
ylabel('y');
grid on;

for k = 1:length(x)
    plot(x(k),y(k),'o', 'Color', colors{k});
    hold on;
end
k = [0:0.1:100];
xt = 10*cos(2*pi*k/200-pi/2);
yt = 10*sin(2*pi*k/200-pi/2) + 10;
plot(xt,yt)
% plot((45:1:75), 1.5, 'x');
% plot((45:1:75), -1.5, 'x');

coder.extrinsic('legend');
legend('a1', 'a2', 'a3', 'a4','a5');

== matlab function Simulink1potradi2/Subsystem/MATLAB Function1 ==
  data: xt input; uax output; yt input; A input; uay output; vx input; vy input
function [uax, uay]= fcn(xt,yt,A, vx, vy)
%funkcija potencijala
uax = zeros(length(A),1);
uay = zeros(length(A),1);
% gainx = zeros(length(A),1);
% gainy = zeros(length(A),1);
% for i = 1:length(A)
%   for j = 1:length(A)
%       if j ~= i
%             gainx(i) = gainx(i) +(xt(i)-xt(j));
%             gainy(i) = gainy(i) + (yt(i)-yt(j));
%       end
%   end
% end

for i = 1:length(A)
  for j = 1:length(A)
      if sqrt((xt(i)-xt(j))^2+(yt(i)-yt(j))^2)<1.5&& j ~= i
            uax(i) = uax(i) + A(i,j)*(1.5/sqrt((xt(i)-xt(j))^2+(yt(i)-yt(j))^2)-1)*1/sqrt((xt(i)-xt(j))^2+(yt(i)-yt(j))^2)^3*(xt(i)-xt(j));
            uay(i) = uay(i) + A(i,j)*(1.5/sqrt((xt(i)-xt(j))^2+(yt(i)-yt(j))^2)-1)*1/sqrt((xt(i)-xt(j))^2+(yt(i)-yt(j))^2)^3*(yt(i)-yt(j));
      end
  end
end

== matlab function Simulink1potradi2/MATLAB Function1 ==
  data: Rt output; R input; t input
function Rt = fcn( R, t)

%T = [cos(atan2(ty,tx)), -sin(atan2(ty,tx));sin(atan2(ty,tx)),cos(atan2(ty,tx))]; % akc-prijelazi

alpha = 2*pi/200*t;
%alpha = 45*pi/180;
%alpha = atan2(2*t/100, 1);

T = [cos(alpha), -sin(alpha);sin(alpha),cos(alpha)];
Rt = T*R;
% Rt = [ 9*cos((u-500)/100), 7*cos((u-500)/100), 5*cos((u-500)/100), 3*cos((u-500)/100), 1*cos((u-500)/100); 9*sin((u-500)/100), 7*sin((u-500)/100), 5*sin((u-500)/100), 3*sin((u-500)/100), 1*sin((u-500)/100)];

== matlab function Simulink1potradi2/MATLAB Function2 ==
  data: G output; t input
function G= fcn(t)

% G = [0 sin(t/100) sin(t/100) sin(t/100) sin(t/100);
%     sin(t/100) 0 cos(t/100) cos(t/100) cos(t/100);
%     sin(t/100) cos(t/100) 0 sin(t/100) sin(t/100);
%     sin(t/100) cos(t/100) sin(t/100) 0 cos(t/100);
%     sin(t/100) cos(t/100) sin(t/100) cos(t/100) 0];
G = [0 1 1 1 1;
    1 0 1 1 1;
    1 1 0 1 1;
    1 1 1 0 1;
    1 1 1 1 0];
G = 0.05*G;
